simulink model "lab_3_task_4_simulink"  (R2025b)
settings: Solver=VariableStepAuto  StartTime=0.0  StopTime=10.0  RelTol=1e-3
values from neighbouring files (symbols this model uses):
  I = diag([0.070 0.055 0.025])    [lab_3_task_4.m]    (also in lab_4_task_1.m = diag([ix iy iz]); lab_5_task_1.m = diag([ix iy iz]); lab_5_task_2.m = diag([ix iy iz]); lab_6_task_1.m = diag([ ix iy iz ]))
  w = simout.w.Data    [lab_3_task_4.m]    (also in lab_5_task_1.m; lab_5_task_2.m; lab_6_task_1.m; lab_6_task_2.m)
libraries: matrix_library x1
settings Model: Creator=User  LastModifiedBy=User

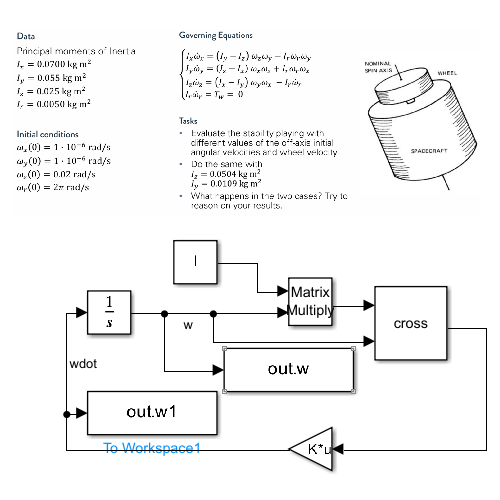
[thumbnail: Simulink's stored preview of the top-level diagram]
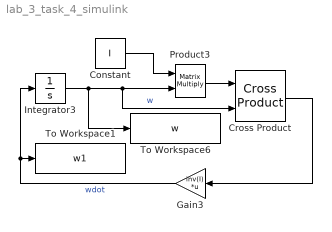
== system lab_3_task_4_simulink ==
  Constant : Constant  Value=I
  Cross Product : matrix_library/Cross Product
  Gain3 : Gain  Gain=inv(I)  Multiplication=Matrix(K*u)
  Integrator3 : Integrator  InitialCondition=w
  Product3 : Product  Multiplication=Matrix(*)
  To Workspace1 : ToWorkspace  VariableName=w1  SaveFormat=Timeseries  SampleTime=-1
  To Workspace6 : ToWorkspace  VariableName=w  SaveFormat=Timeseries  SampleTime=-1
  wires:
  Constant/1 -> Product3/1
  Gain3/1 -> Integrator3/1, To Workspace1/1  "wdot"
  Product3/1 -> Cross Product/1
  Integrator3/1 -> To Workspace6/1, Cross Product/2, Product3/2  "w"
  Cross Product/1 -> Gain3/1
